simulink model "slm4"  (R2018a)
settings: Solver=VariableStepAuto  StartTime=0.0  StopTime=10.0  RelTol=1e-3
values from neighbouring files (symbols this model uses):
  c1 = 116    [setup.m]
  k1 = 3930    [setup.m]
  k2 = 5720    [setup.m]
  X = 1    [setup.m]
settings Model: Creator=Pranav Maddula  LastModifiedBy=Pranav Maddula

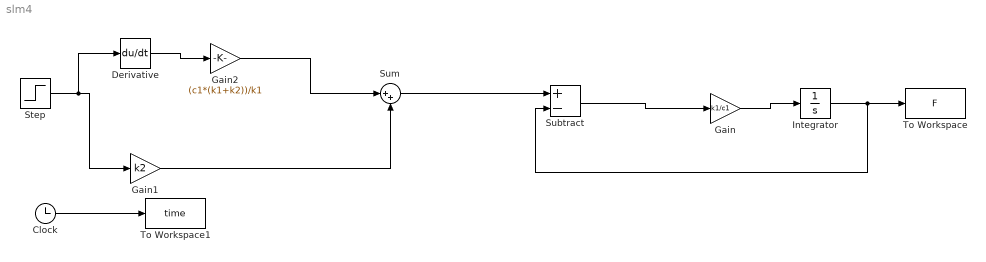
== system slm4 ==
  Clock : Clock
  Derivative : Derivative
  Gain : Gain  Gain=k1/c1
  Gain1 : Gain  Gain=k2
  Gain2 : Gain  Gain=(c1*(k1+k2))/k1
  Integrator : Integrator
  Step : Step  After=X  SampleTime=0
  Subtract : Sum  Inputs=+-
  Sum : Sum  Inputs=|++
  To Workspace : ToWorkspace  VariableName=F  SampleTime=-1
  To Workspace1 : ToWorkspace  VariableName=time  SampleTime=-1
  wires:
  Integrator/1 -> Subtract/2, To Workspace/1
  Gain/1 -> Integrator/1
  Subtract/1 -> Gain/1
  Sum/1 -> Subtract/1
  Step/1 -> Derivative/1, Gain1/1
  Gain1/1 -> Sum/2
  Derivative/1 -> Gain2/1
  Gain2/1 -> Sum/1
  Clock/1 -> To Workspace1/1
